simulink model "No_Guide_Experiments"  (R2020b)
settings: Solver=FixedStepAuto  StartTime=0.0  StopTime=1400  FixedStep=1  RelTol=1e-3  AbsTol=1e-6
model workspace (MATLAB code in the model file):
  | % load initial conditions and physical properties from file
  | 
  | data;
values from neighbouring files (symbols this model uses):
  c = 1005.4    [data.m]
  densAir = 1.2250    (= 1.225)    [data.m]
  M = (lenHouse*widHouse*htHouse+tan(pitRoof)*widHouse*lenHouse)*densAir    [data.m]
  Mdot = 60    [data.m]
  Req = RWall*RWindow/(RWall + RWindow)    [data.m]
libraries: dspnetwork x2
settings Model: ExtModeTrigMode=oneshot  ExtModeArmWhenConnect=off  ExtModeAutoUpdateStatusClock=off  OrderedModelArguments=off  Creator=The MathWorks, Inc.  LastModifiedBy=xinbo
settings SolverCC: AutoScaleAbsTol=off
settings DataIOCC: ExternalInput=[]  InitialState=[]  SaveFormat=Array  SaveOutput=off  SaveTime=off  SignalLoggingName=sldemo_househeat_output
settings OptimizationCC: BlockReduction=off  BooleanDataType=off  ExpressionDepthLimit=2147483647  InitFltsAndDblsToZero=on  LifeSpan=inf  BufferReusableBoundary=off
settings DebuggingCC: SaveWithParameterizedLinksMsg=none  UnderspecifiedInitializationDetection=Classic  MergeDetectMultiDrivingBlocksExec=none  SignalResolutionControl=TryResolveAllWithWarning  MultiTaskDSMMsg=warning  MultiTaskCondExecSysMsg=none  IntegerOverflowMsg=none  FcnCallInpInsideContextMsg=warning  BusObjectLabelMismatch=none  StateNameClashWarn=warning  SFUnexpectedBacktrackingDiag=warning  SFNoUnconditionalDefaultTransitionDiag=warning  SFExecutionAtInitializationDiag=none  IntegerSaturationMsg=none  ArithmeticOperatorsInVariantConditions=warning
settings HardwareCC: ProdBitPerPointer=32  ProdBitPerSizeT=32  ProdBitPerPtrDiffT=32  ProdLargestAtomicFloat=None  ProdIntDivRoundTo=Undefined  ProdEndianess=Unspecified  ProdWordSize=32  ProdHWDeviceType=32-bit Generic  TargetUnknown=on
settings ModelReferenceCC: PropagateSignalLabelsOutOfModel=off
settings SFSimCC: SimUseLocalCustomCode=off  CustomCodeUndefinedFunction=UseInterfaceOnly
settings RTWCC: RTWUseLocalCustomCode=off
settings CodeAppCC: StateflowObjectComments=on
settings GRTTargetCC: TargetFcnLib=ansi_tfl_tmw.mat  TargetLangStandard=C89/C90 (ANSI)  CombineOutputUpdateFcns=off  GRTInterface=on
settings ConfigComp: CovMetricSettings=dw  CovSaveCumulativeToWorkspaceVar=on  CovSaveSingleToWorkspaceVar=on  CovExternalEMLEnable=off

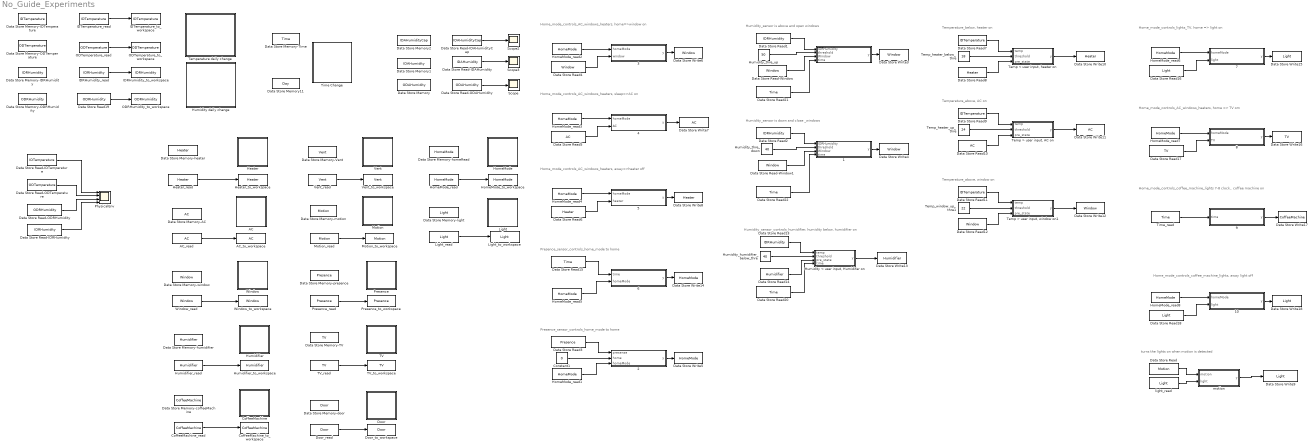
== system No_Guide_Experiments ==
  note: Home_mode_controls_coffee_machine_lights 7-8 clock,. coffee machine on
  note: Humidity_sensor is down and close _windows
  note: Home_mode_controls_AC_windows_heaters, home => TV om
  note: Temperature_below, heater on
  note: Home_mode_controls_lights_TV, home => light on
  note: Presence_sensor_controls_home_mode to home
  note: Presence_sensor_controls_home_mode to home
  note: Humidity_sensor_controls_humidifier, humidity below, humidifier on
  note: Temperature_above, window on
  note: Home_mode_controls_coffee_machine_lights, away light off
  note: Temperature_above, AC on
  note: Home_mode_controls_AC_windows_heaters, sleep=>AC on
  note: turns the lights on when motion is detected
  note: Home_mode_controls_AC_windows_heaters, away=>heater off
  note: Home_mode_controls_AC_windows_heaters, home=>window on
  note: Humidity_sensor is above and open windows
  " " : MATLAB Function  TreatAsAtomicUnit=on
  " 1" : MATLAB Function  TreatAsAtomicUnit=on
  " 10" : MATLAB Function  TreatAsAtomicUnit=on
  " 2" : MATLAB Function  TreatAsAtomicUnit=on
  " 3" : MATLAB Function  TreatAsAtomicUnit=on
  " 4" : MATLAB Function  TreatAsAtomicUnit=on
  " 5" : MATLAB Function  TreatAsAtomicUnit=on
  " 6" : MATLAB Function  TreatAsAtomicUnit=on
  " 7" : MATLAB Function  TreatAsAtomicUnit=on
  " 8" : MATLAB Function  TreatAsAtomicUnit=on
  " 9" : MATLAB Function  TreatAsAtomicUnit=on
  AC : Subsystem
      mask Display: image('$imagefile'); % Use "Edit Image" on toolstrip to change.
  AC_read : DataStoreRead  DataStoreName=AC
  AC_to_workspace : ToWorkspace  VariableName=AC  SampleTime=-1
      settings: Save2DSignal=2-D array (concatenate along first dimension)
  CoffeeMachine : Subsystem
      mask Display: image('$imagefile'); % Use "Edit Image" on toolstrip to change.
  CoffeeMachine_read : DataStoreRead  DataStoreName=CoffeeMachine
  CoffeeMachine_to_workspace : ToWorkspace  VariableName=CoffeeMachine  SampleTime=-1
      settings: Save2DSignal=2-D array (concatenate along first dimension)
  Constant1 : Constant  Value=0
  Data Store Memory11 : DataStoreMemory  DataStoreName=Day  ReadBeforeWriteMsg=warning  WriteAfterWriteMsg=warning  WriteAfterReadMsg=warning  ShowAdditionalParam=off  OutDataTypeStr=double
  Data Store Read : DataStoreRead  DataStoreName=Motion
  Data Store Read-IDAHumidity : DataStoreRead  DataStoreName=IDAHumidity
  Data Store Read-IDAHumidityCap : DataStoreRead  DataStoreName=IDAHumidityCap
  Data Store Read-IDRHumidity : DataStoreRead  DataStoreName=IDRHumidity
  Data Store Read-IDTemperature : DataStoreRead  DataStoreName=IDTemperature
  Data Store Read-ODAHumidity : DataStoreRead  DataStoreName=ODAHumidity
  Data Store Read-ODRHumidity : DataStoreRead  DataStoreName=ODRHumidity
  Data Store Read-ODTemperature : DataStoreRead  DataStoreName=ODTemperature
  Data Store Read1 : DataStoreRead  DataStoreName=IDRHumidity
  Data Store Read10 : DataStoreRead  DataStoreName=AC
  Data Store Read11 : DataStoreRead  DataStoreName=IDTemperature
  Data Store Read12 : DataStoreRead  DataStoreName=Window
  Data Store Read13 : DataStoreRead  DataStoreName=IDRHumidity
  Data Store Read14 : DataStoreRead  DataStoreName=Humidifier
  Data Store Read{15,20..22} (4 alike) : DataStoreRead  DataStoreName=Time
  Data Store Read16 : DataStoreRead  DataStoreName=Light
  Data Store Read17 : DataStoreRead  DataStoreName=TV
  Data Store Read18 : DataStoreRead  DataStoreName=Light
  Data Store Read19 : DataStoreRead  DataStoreName=ODRHumidity
  Data Store Read2 : DataStoreRead  DataStoreName=IDRHumidity
  Data Store Read3 : DataStoreRead  DataStoreName=Presence
  Data Store Read4 : DataStoreRead  DataStoreName=Window
  Data Store Read5 : DataStoreRead  DataStoreName=AC
  Data Store Read6 : DataStoreRead  DataStoreName=Heater
  Data Store Read7 : DataStoreRead  DataStoreName=IDTemperature
  Data Store Read8 : DataStoreRead  DataStoreName=Heater
  Data Store Read9 : DataStoreRead  DataStoreName=IDTemperature
  Data Store Write10 : DataStoreWrite  DataStoreName=Heater
  Data Store Write11 : DataStoreWrite  DataStoreName=AC
  Data Store Write{3..4,6,12} (4 alike) : DataStoreWrite  DataStoreName=Window
  Data Store Write13 : DataStoreWrite  DataStoreName=Humidifier
  Data Store Write14 : DataStoreWrite  DataStoreName=HomeMode
  Data Store Write15 : DataStoreWrite  DataStoreName=Light
  Data Store Write16 : DataStoreWrite  DataStoreName=TV
  Data Store Write17 : DataStoreWrite  DataStoreName=CoffeeMachine
  Data Store Write18 : DataStoreWrite  DataStoreName=Light
  Data Store Write5 : DataStoreWrite  DataStoreName=HomeMode
  Data Store Write7 : DataStoreWrite  DataStoreName=AC
  Data Store Write8 : DataStoreWrite  DataStoreName=Heater
  Data Store Write9 : DataStoreWrite  DataStoreName=Light
  Data Store Memory : DataStoreMemory  DataStoreName=ODAHumidity  ReadBeforeWriteMsg=warning  WriteAfterWriteMsg=warning  WriteAfterReadMsg=warning  ShowAdditionalParam=off
  Data Store Memory-AC : DataStoreMemory  DataStoreName=AC  ReadBeforeWriteMsg=warning  WriteAfterWriteMsg=warning  WriteAfterReadMsg=warning  ShowAdditionalParam=off  OutDataTypeStr=double
  Data Store Memory-IDRHumidity : DataStoreMemory  DataStoreName=IDRHumidity  ReadBeforeWriteMsg=warning  WriteAfterWriteMsg=warning  WriteAfterReadMsg=warning  InitialValue=80  ShowAdditionalParam=off  OutDataTypeStr=double
  Data Store Memory-IDTemperature : DataStoreMemory  DataStoreName=IDTemperature  ReadBeforeWriteMsg=warning  WriteAfterWriteMsg=warning  WriteAfterReadMsg=warning  InitialValue=25  ShowAdditionalParam=off  OutDataTypeStr=double
  Data Store Memory-ODRHumidity : DataStoreMemory  DataStoreName=ODRHumidity  ReadBeforeWriteMsg=warning  WriteAfterWriteMsg=warning  WriteAfterReadMsg=warning  InitialValue=45  ShowAdditionalParam=off  OutDataTypeStr=double
  Data Store Memory-ODTemperature : DataStoreMemory  DataStoreName=ODTemperature  ReadBeforeWriteMsg=warning  WriteAfterWriteMsg=warning  WriteAfterReadMsg=warning  ShowAdditionalParam=off  OutDataTypeStr=double
  Data Store Memory-TV : DataStoreMemory  DataStoreName=TV  ReadBeforeWriteMsg=warning  WriteAfterWriteMsg=warning  WriteAfterReadMsg=warning  ShowAdditionalParam=off  OutDataTypeStr=double
  Data Store Memory-Time : DataStoreMemory  DataStoreName=Time  ReadBeforeWriteMsg=warning  WriteAfterWriteMsg=warning  WriteAfterReadMsg=warning  ShowAdditionalParam=off  OutDataTypeStr=double
  Data Store Memory-Vent : DataStoreMemory  DataStoreName=Vent  ReadBeforeWriteMsg=warning  WriteAfterWriteMsg=warning  WriteAfterReadMsg=warning  ShowAdditionalParam=off
  Data Store Memory-coffeeMachine : DataStoreMemory  DataStoreName=CoffeeMachine  ReadBeforeWriteMsg=warning  WriteAfterWriteMsg=warning  WriteAfterReadMsg=warning  ShowAdditionalParam=off
  Data Store Memory-door : DataStoreMemory  DataStoreName=Door  ReadBeforeWriteMsg=warning  WriteAfterWriteMsg=warning  WriteAfterReadMsg=warning  ShowAdditionalParam=off  OutDataTypeStr=int8
  Data Store Memory-heater : DataStoreMemory  DataStoreName=Heater  ReadBeforeWriteMsg=warning  WriteAfterWriteMsg=warning  WriteAfterReadMsg=warning  ShowAdditionalParam=off
  Data Store Memory-homeRead : DataStoreMemory  DataStoreName=HomeMode  ReadBeforeWriteMsg=warning  WriteAfterWriteMsg=warning  WriteAfterReadMsg=warning  InitialValue=2  ShowAdditionalParam=off  OutDataTypeStr=double
  Data Store Memory-humidifier : DataStoreMemory  DataStoreName=Humidifier  ReadBeforeWriteMsg=warning  WriteAfterWriteMsg=warning  WriteAfterReadMsg=warning  ShowAdditionalParam=off
  Data Store Memory-light : DataStoreMemory  DataStoreName=Light  ReadBeforeWriteMsg=warning  WriteAfterWriteMsg=warning  WriteAfterReadMsg=warning  ShowAdditionalParam=off  OutDataTypeStr=double
  Data Store Memory-motion : DataStoreMemory  DataStoreName=Motion  ReadBeforeWriteMsg=warning  WriteAfterWriteMsg=warning  WriteAfterReadMsg=warning  ShowAdditionalParam=off
  Data Store Memory-presence : DataStoreMemory  DataStoreName=Presence  ReadBeforeWriteMsg=warning  WriteAfterWriteMsg=warning  WriteAfterReadMsg=warning  ShowAdditionalParam=off
  Data Store Memory-window : DataStoreMemory  DataStoreName=Window  ReadBeforeWriteMsg=warning  WriteAfterWriteMsg=warning  WriteAfterReadMsg=warning  ShowAdditionalParam=off
  Data Store Memory1 : DataStoreMemory  DataStoreName=IDAHumidity  ReadBeforeWriteMsg=warning  WriteAfterWriteMsg=warning  WriteAfterReadMsg=warning  ShowAdditionalParam=off
  Data Store Memory2 : DataStoreMemory  DataStoreName=IDAHumidityCap  ReadBeforeWriteMsg=warning  WriteAfterWriteMsg=warning  WriteAfterReadMsg=warning  ShowAdditionalParam=off
  Data Store Read-Window : DataStoreRead  DataStoreName=Window
  Data Store Read-Window1 : DataStoreRead  DataStoreName=Window
  Door : Subsystem
      mask Display: image('$imagefile'); % Use "Edit Image" on toolstrip to change.
  Door_read : DataStoreRead  DataStoreName=Door
  Door_to_workspace : ToWorkspace  VariableName=Door  SampleTime=-1
      settings: Save2DSignal=2-D array (concatenate along first dimension)
  Heater : Subsystem
      mask Display: image('$imagefile'); % Use "Edit Image" on toolstrip to change.
  Heater_read : DataStoreRead  DataStoreName=Heater
  Heater_to_workspace : ToWorkspace  VariableName=Heater  SampleTime=-1
      settings: Save2DSignal=2-D array (concatenate along first dimension)
  HomeMode : Subsystem
      mask Display: image('$imagefile'); % Use "Edit Image" on toolstrip to change.
  HomeMode_read{,1..8} (9 alike) : DataStoreRead  DataStoreName=HomeMode
  HomeMode_to_workspace : ToWorkspace  VariableName=HomeMode  SampleTime=-1
      settings: Save2DSignal=2-D array (concatenate along first dimension)
  Humidifier : Subsystem
      mask Display: image('$imagefile'); % Use "Edit Image" on toolstrip to change.
  Humidifier_read : DataStoreRead  DataStoreName=Humidifier
  Humidifier_to_workspace : ToWorkspace  VariableName=Humidifier  SampleTime=-1
      settings: Save2DSignal=2-D array (concatenate along first dimension)
  "Humidity < user input, Humidifer on" : MATLAB Function  TreatAsAtomicUnit=on
  Humidity daily change : Subsystem
      mask Display: image('$imagefile'); % Use "Edit Image" on toolstrip to change.
  Humidity_humidifier_below_thre : Constant  Value=40
  Humidity_thre_down : Constant  Value=40
  Humidity_thre_up : Constant  Value=50
  IDRHumidity_read : DataStoreRead  DataStoreName=IDRHumidity
  IDRHumidity_to_workspace : ToWorkspace  VariableName=IDRHumidity  SampleTime=-1
      settings: Save2DSignal=2-D array (concatenate along first dimension)
  IDTemperature_read : DataStoreRead  DataStoreName=IDTemperature
  IDTemperature_to_workspace : ToWorkspace  VariableName=IDTemperature  SampleTime=-1
      settings: Save2DSignal=2-D array (concatenate along first dimension)
  Light : Subsystem
      mask Display: image('$imagefile'); % Use "Edit Image" on toolstrip to change.
  Light_read : DataStoreRead  DataStoreName=Light
  Light_to_workspace : ToWorkspace  VariableName=Light  SampleTime=-1
      settings: Save2DSignal=2-D array (concatenate along first dimension)
  Motion : Subsystem
      mask Display: image('$imagefile'); % Use "Edit Image" on toolstrip to change.
  Motion_read : DataStoreRead  DataStoreName=Motion
  Motion_to_workspace : ToWorkspace  VariableName=Motion  SampleTime=-1
      settings: Save2DSignal=2-D array (concatenate along first dimension)
  ODRHumidity_to_workspace : ToWorkspace  VariableName=ODRHumidity  SampleTime=-1
      settings: Save2DSignal=2-D array (concatenate along first dimension)
  ODTemperature_read : DataStoreRead  DataStoreName=ODTemperature
  ODTemperature_to_workspace : ToWorkspace  VariableName=ODTemperature  SampleTime=-1
      settings: Save2DSignal=2-D array (concatenate along first dimension)
  PhysicalEnv : Scope  NumInputPorts=4
  Presence : Subsystem
      mask Display: image('$imagefile'); % Use "Edit Image" on toolstrip to change.
  Presence_read : DataStoreRead  DataStoreName=Presence
  Presence_to_workspace : ToWorkspace  VariableName=Presence  SampleTime=-1
      settings: Save2DSignal=2-D array (concatenate along first dimension)
  Scope : Scope
  Scope2 : Scope
  Scope3 : Scope
  TV : Subsystem
      mask Display: image('$imagefile'); % Use "Edit Image" on toolstrip to change.
  TV_read : DataStoreRead  DataStoreName=TV
  TV_to_workspace : ToWorkspace  VariableName=TV  SampleTime=-1
      settings: Save2DSignal=2-D array (concatenate along first dimension)
  "Temp < user input, heater on" : MATLAB Function  TreatAsAtomicUnit=on
  "Temp > user input, AC on" : MATLAB Function  TreatAsAtomicUnit=on
  "Temp > user input, window on1" : MATLAB Function  TreatAsAtomicUnit=on
  Temp_heater_below_thre : Constant  Value=18
  Temp_heater_up_thre : Constant  Value=24
  Temp_window_up_thre1 : Constant  Value=22
  Temperature daily change : Subsystem
      mask Display: image('$imagefile'); % Use "Edit Image" on toolstrip to change.
  Time Change : Subsystem
      mask Display: image('$imagefile'); % Use "Edit Image" on toolstrip to change.
  Time_read : DataStoreRead  DataStoreName=Time
  Vent : Subsystem
      mask Display: image('$imagefile'); % Use "Edit Image" on toolstrip to change.
  Vent_read : DataStoreRead  DataStoreName=Vent
  Vent_to_workspace : ToWorkspace  VariableName=Vent  SampleTime=-1
      settings: Save2DSignal=2-D array (concatenate along first dimension)
  Window : Subsystem
      mask Display: image('$imagefile'); % Use "Edit Image" on toolstrip to change.
  Window_read : DataStoreRead  DataStoreName=Window
  Window_to_workspace : ToWorkspace  VariableName=Window  SampleTime=-1
      settings: Save2DSignal=2-D array (concatenate along first dimension)
  light_read : DataStoreRead  DataStoreName=Light  SampleTime=1
  motion : MATLAB Function  TreatAsAtomicUnit=on
  wires:
  Temp_heater_up_thre/1 -> "Temp > user input, AC on"/2(threshold)
  Data Store Read21/1 -> " "/4(time)
  Data Store Read3/1 -> " 2"/1(presense)
  light_read/1 -> motion/2(light)
  " 10"/1(y) -> Data Store Write18/1
  motion/1(y) -> Data Store Write9/1
  " 4"/1(y) -> Data Store Write7/1
  Data Store Read-Window1/1 -> " 1"/3(Window)
  Humidity_thre_down/1 -> " 1"/2(threshold)
  HomeMode_read3/1 -> " 4"/1(homeMode)
  "Humidity < user input, Humidifer on"/1(y) -> Data Store Write13/1
  Data Store Read12/1 -> "Temp > user input, window on1"/3(pre_state)
  Data Store Read15/1 -> " 6"/1(time)
  " 2"/1(y) -> Data Store Write5/1
  HomeMode_read5/1 -> " 6"/2(homeMode)
  Data Store Read/1 -> motion/1(motion)
  Constant1/1 -> " 2"/2(home)
  Data Store Read6/1 -> " 5"/2(heater)
  Data Store Read11/1 -> "Temp > user input, window on1"/1(temp)
  " 5"/1(y) -> Data Store Write8/1
  Data Store Read16/1 -> " 7"/2(light)
  "Temp > user input, AC on"/1(y) -> Data Store Write11/1
  " "/1(y) -> Data Store Write3/1
  Data Store Read14/1 -> "Humidity < user input, Humidifer on"/3(pre_state)
  HomeMode_read4/1 -> " 5"/1(homeMode)
  HomeMode_read2/1 -> " 3"/1(homeMode)
  "Temp > user input, window on1"/1(y) -> Data Store Write12/1
  Data Store Read2/1 -> " 1"/1(IDRHumidity)
  HomeMode_read1/1 -> " 2"/3(homeMode)
  Data Store Read4/1 -> " 3"/2(window)
  Temp_heater_below_thre/1 -> "Temp < user input, heater on"/2(threshold)
  Data Store Read9/1 -> "Temp > user input, AC on"/1(temp)
  Temp_window_up_thre1/1 -> "Temp > user input, window on1"/2(threshold)
  " 3"/1(y) -> Data Store Write6/1
  Data Store Read1/1 -> " "/1(IDRHumidity)
  Data Store Read17/1 -> " 8"/2(TV)
  HomeMode_read6/1 -> " 7"/1(homeMode)
  Data Store Read7/1 -> "Temp < user input, heater on"/1(temp)
  Data Store Read10/1 -> "Temp > user input, AC on"/3(pre_state)
  HomeMode_read7/1 -> " 8"/1(homeMode)
  Time_read/1 -> " 9"/1(time)
  Data Store Read-Window/1 -> " "/3(Window)
  Data Store Read5/1 -> " 4"/2(AC)
  " 1"/1(y) -> Data Store Write4/1
  HomeMode_read8/1 -> " 10"/1(homeMode)
  Data Store Read8/1 -> "Temp < user input, heater on"/3(pre_state)
  "Temp < user input, heater on"/1(y) -> Data Store Write10/1
  Data Store Read13/1 -> "Humidity < user input, Humidifer on"/1(temp)
  Humidity_thre_up/1 -> " "/2(threshold)
  " 7"/1(y) -> Data Store Write15/1
  Data Store Read18/1 -> " 10"/2(light)
  " 9"/1(y) -> Data Store Write17/1
  " 8"/1(y) -> Data Store Write16/1
  Data Store Read20/1 -> "Humidity < user input, Humidifer on"/4(time)
  Humidity_humidifier_below_thre/1 -> "Humidity < user input, Humidifer on"/2(threshold)
  " 6"/1(y) -> Data Store Write14/1
  Data Store Read22/1 -> " 1"/4(time)
  Data Store Read-ODAHumidity/1 -> Scope/1
  Data Store Read-ODTemperature/1 -> PhysicalEnv/2
  Motion_read/1 -> Motion_to_workspace/1
  Data Store Read-IDRHumidity/1 -> PhysicalEnv/4
  Heater_read/1 -> Heater_to_workspace/1
  Vent_read/1 -> Vent_to_workspace/1
  Door_read/1 -> Door_to_workspace/1
  Data Store Read-IDTemperature/1 -> PhysicalEnv/1
  Window_read/1 -> Window_to_workspace/1
  Humidifier_read/1 -> Humidifier_to_workspace/1
  CoffeeMachine_read/1 -> CoffeeMachine_to_workspace/1
  IDRHumidity_read/1 -> IDRHumidity_to_workspace/1
  Data Store Read-IDAHumidityCap/1 -> Scope2/1
  Data Store Read-IDAHumidity/1 -> Scope3/1
  Data Store Read-ODRHumidity/1 -> PhysicalEnv/3
  Presence_read/1 -> Presence_to_workspace/1
  IDTemperature_read/1 -> IDTemperature_to_workspace/1
  TV_read/1 -> TV_to_workspace/1
  ODTemperature_read/1 -> ODTemperature_to_workspace/1
  Light_read/1 -> Light_to_workspace/1
  AC_read/1 -> AC_to_workspace/1
  Data Store Read19/1 -> ODRHumidity_to_workspace/1
  HomeMode_read/1 -> HomeMode_to_workspace/1

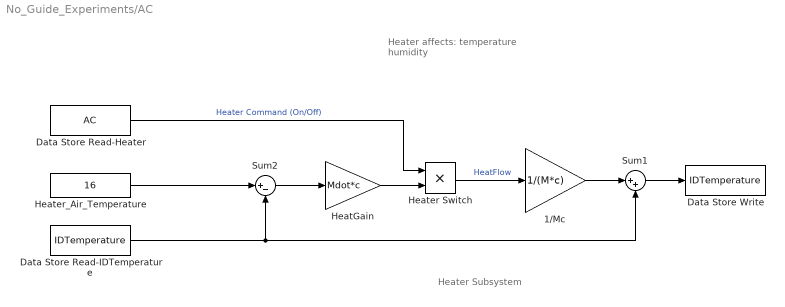
== system No_Guide_Experiments/AC ==
  note: Heater affects:
      | temperature
      | humidity
  note: Heater Subsystem
  1/Mc : Gain  Gain=1/(M*c)  SaturateOnIntegerOverflow=on  OutDataTypeStr=Inherit: Same as input  ParamDataTypeStr=Inherit: Same as input
  Data Store Read-Heater : DataStoreRead  DataStoreName=AC
  Data Store Read-IDTemperature : DataStoreRead  DataStoreName=IDTemperature
  Data Store Write : DataStoreWrite  DataStoreName=IDTemperature
  HeatGain : Gain  Gain=Mdot*c
  Heater Switch : Product  RndMeth=Zero
  Heater_Air_Temperature : Constant  Value=16
  Sum1 : Sum  Inputs=|++  InputSameDT=on  SaturateOnIntegerOverflow=on  OutDataTypeStr=Inherit: Same as first input
  Sum2 : Sum  Inputs=|+-
  wires:
  Data Store Read-Heater/1 -> Heater Switch/1  "Heater Command (On/Off)"
  Sum2/1 -> HeatGain/1
  Heater_Air_Temperature/1 -> Sum2/1
  HeatGain/1 -> Heater Switch/2
  Heater Switch/1 -> 1/Mc/1  "HeatFlow"
  1/Mc/1 -> Sum1/1
  Data Store Read-IDTemperature/1 -> Sum1/2, Sum2/2
  Sum1/1 -> Data Store Write/1

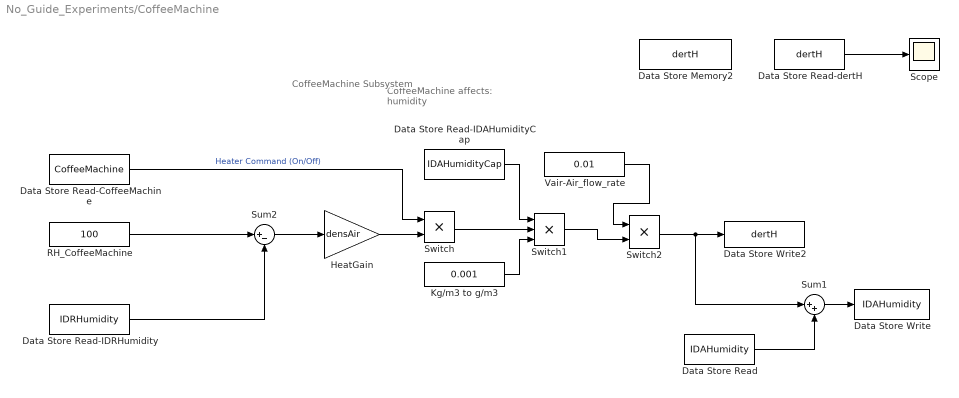
== system No_Guide_Experiments/CoffeeMachine ==
  note: CoffeeMachine affects:
      | humidity
  note: CoffeeMachine
      |  Subsystem
  " Switch" : Product  RndMeth=Zero
  " Switch1" : Product  Inputs=3  RndMeth=Zero
  " Switch2" : Product  RndMeth=Zero
  Data Store Read : DataStoreRead  DataStoreName=IDAHumidity
  Data Store Read-CoffeeMachine : DataStoreRead  DataStoreName=CoffeeMachine
  Data Store Read-IDAHumidityCap : DataStoreRead  DataStoreName=IDAHumidityCap
  Data Store Read-IDRHumidity : DataStoreRead  DataStoreName=IDRHumidity
  Data Store Read-dertH : DataStoreRead  DataStoreName=dertH
  Data Store Write : DataStoreWrite  DataStoreName=IDAHumidity
  Data Store Write2 : DataStoreWrite  DataStoreName=dertH
  Data Store Memory2 : DataStoreMemory  DataStoreName=dertH  ReadBeforeWriteMsg=warning  WriteAfterWriteMsg=warning  WriteAfterReadMsg=warning  ShowAdditionalParam=off
  HeatGain : Gain  Gain=densAir
  Kg/m3 to g/m3 : Constant  Value=0.001
  RH_CoffeeMachine : Constant  Value=100
  Scope : Scope
  Sum1 : Sum  Inputs=|++
  Sum2 : Sum  Inputs=|+-
  Vair-Air_flow_rate : Constant  Value=0.01
  wires:
  Data Store Read-CoffeeMachine/1 -> " Switch"/1  "Heater Command (On/Off)"
  Sum2/1 -> HeatGain/1
  RH_CoffeeMachine/1 -> Sum2/1
  HeatGain/1 -> " Switch"/2
  " Switch"/1 -> " Switch1"/2
  Data Store Read-IDRHumidity/1 -> Sum2/2
  Data Store Read-IDAHumidityCap/1 -> " Switch1"/1
  Kg/m3 to g/m3/1 -> " Switch1"/3
  " Switch1"/1 -> " Switch2"/2
  Vair-Air_flow_rate/1 -> " Switch2"/1
  " Switch2"/1 -> Sum1/1, Data Store Write2/1
  Sum1/1 -> Data Store Write/1
  Data Store Read-dertH/1 -> Scope/1
  Data Store Read/1 -> Sum1/2

== system No_Guide_Experiments/Door ==

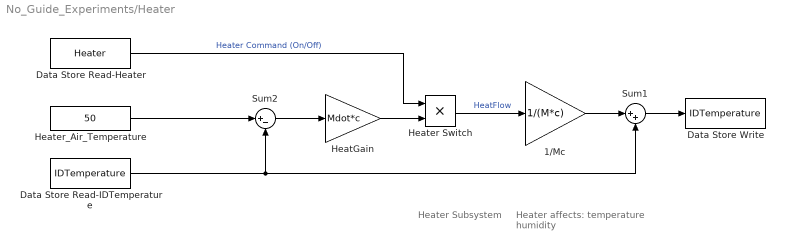
== system No_Guide_Experiments/Heater ==
  note: Heater affects:
      | temperature
      | humidity
  note: Heater Subsystem
  1/Mc : Gain  Gain=1/(M*c)  SaturateOnIntegerOverflow=on  OutDataTypeStr=Inherit: Same as input  ParamDataTypeStr=Inherit: Same as input
  Data Store Read-Heater : DataStoreRead  DataStoreName=Heater
  Data Store Read-IDTemperature : DataStoreRead  DataStoreName=IDTemperature
  Data Store Write : DataStoreWrite  DataStoreName=IDTemperature
  HeatGain : Gain  Gain=Mdot*c
  Heater Switch : Product  RndMeth=Zero
  Heater_Air_Temperature : Constant  Value=50
  Sum1 : Sum  Inputs=|++  InputSameDT=on  SaturateOnIntegerOverflow=on  OutDataTypeStr=Inherit: Same as first input
  Sum2 : Sum  Inputs=|+-
  wires:
  Data Store Read-Heater/1 -> Heater Switch/1  "Heater Command (On/Off)"
  Sum2/1 -> HeatGain/1
  Heater_Air_Temperature/1 -> Sum2/1
  HeatGain/1 -> Heater Switch/2
  Heater Switch/1 -> 1/Mc/1  "HeatFlow"
  1/Mc/1 -> Sum1/1
  Data Store Read-IDTemperature/1 -> Sum1/2, Sum2/2
  Sum1/1 -> Data Store Write/1

== system No_Guide_Experiments/HomeMode ==

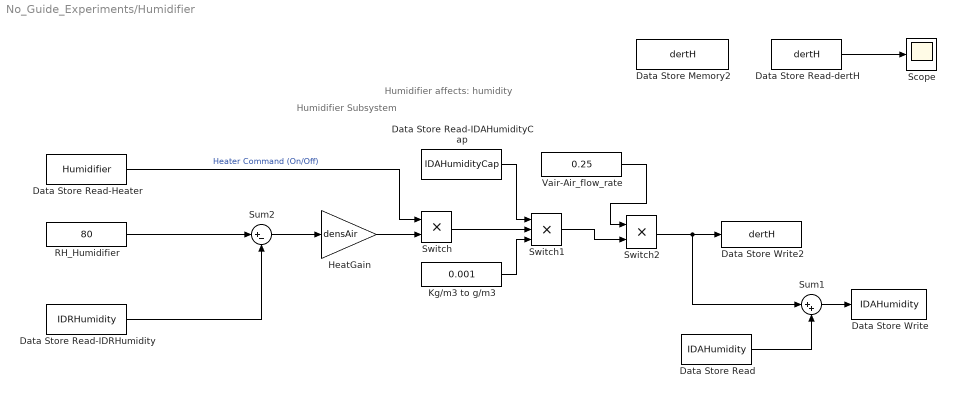
== system No_Guide_Experiments/Humidifier ==
  note: Humidifier affects:
      | humidity
  note: Humidifier
      |  Subsystem
  " Switch" : Product  RndMeth=Zero
  " Switch1" : Product  Inputs=3  RndMeth=Zero
  " Switch2" : Product  RndMeth=Zero
  Data Store Read : DataStoreRead  DataStoreName=IDAHumidity
  Data Store Read-Heater : DataStoreRead  DataStoreName=Humidifier
  Data Store Read-IDAHumidityCap : DataStoreRead  DataStoreName=IDAHumidityCap
  Data Store Read-IDRHumidity : DataStoreRead  DataStoreName=IDRHumidity
  Data Store Read-dertH : DataStoreRead  DataStoreName=dertH
  Data Store Write : DataStoreWrite  DataStoreName=IDAHumidity
  Data Store Write2 : DataStoreWrite  DataStoreName=dertH
  Data Store Memory2 : DataStoreMemory  DataStoreName=dertH  ReadBeforeWriteMsg=warning  WriteAfterWriteMsg=warning  WriteAfterReadMsg=warning  ShowAdditionalParam=off
  HeatGain : Gain  Gain=densAir
  Kg/m3 to g/m3 : Constant  Value=0.001
  RH_Humidifier : Constant  Value=80
  Scope : Scope
  Sum1 : Sum  Inputs=|++
  Sum2 : Sum  Inputs=|+-
  Vair-Air_flow_rate : Constant  Value=0.25
  wires:
  Data Store Read-Heater/1 -> " Switch"/1  "Heater Command (On/Off)"
  Sum2/1 -> HeatGain/1
  RH_Humidifier/1 -> Sum2/1
  HeatGain/1 -> " Switch"/2
  " Switch"/1 -> " Switch1"/2
  Data Store Read-IDRHumidity/1 -> Sum2/2
  Data Store Read-IDAHumidityCap/1 -> " Switch1"/1
  Kg/m3 to g/m3/1 -> " Switch1"/3
  " Switch1"/1 -> " Switch2"/2
  Vair-Air_flow_rate/1 -> " Switch2"/1
  " Switch2"/1 -> Sum1/1, Data Store Write2/1
  Sum1/1 -> Data Store Write/1
  Data Store Read-dertH/1 -> Scope/1
  Data Store Read/1 -> Sum1/2

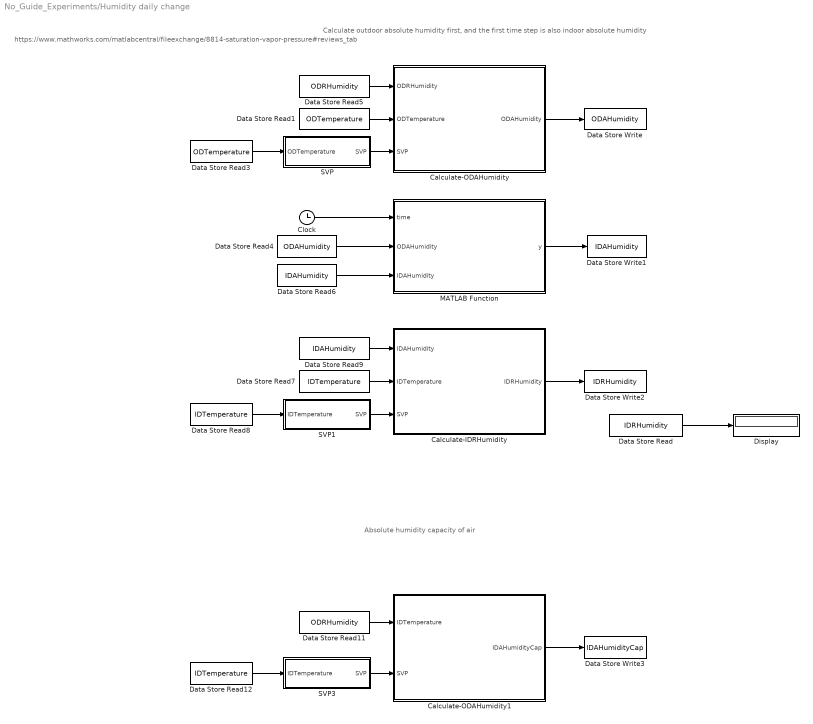
== system No_Guide_Experiments/Humidity daily change ==
  note: Absolute humidity capacity of air
  note: https://www.mathworks.com/matlabcentral/fileexchange/8814-saturation-vapor-pressure#reviews_tab
  note: Calculate outdoor absolute humidity first, and the first time step is also indoor absolute humidity
  Calculate-IDRHumidity : MATLAB Function  TreatAsAtomicUnit=on
  Calculate-ODAHumidity : MATLAB Function  TreatAsAtomicUnit=on
  Calculate-ODAHumidity1 : MATLAB Function  TreatAsAtomicUnit=on
  Clock : Clock
  Data Store Read : DataStoreRead  DataStoreName=IDRHumidity
  Data Store Read1 : DataStoreRead  DataStoreName=ODTemperature
  Data Store Read11 : DataStoreRead  DataStoreName=ODRHumidity
  Data Store Read12 : DataStoreRead  DataStoreName=IDTemperature
  Data Store Read3 : DataStoreRead  DataStoreName=ODTemperature
  Data Store Read4 : DataStoreRead  DataStoreName=ODAHumidity
  Data Store Read5 : DataStoreRead  DataStoreName=ODRHumidity
  Data Store Read6 : DataStoreRead  DataStoreName=IDAHumidity
  Data Store Read7 : DataStoreRead  DataStoreName=IDTemperature
  Data Store Read8 : DataStoreRead  DataStoreName=IDTemperature
  Data Store Read9 : DataStoreRead  DataStoreName=IDAHumidity
  Data Store Write : DataStoreWrite  DataStoreName=ODAHumidity
  Data Store Write1 : DataStoreWrite  DataStoreName=IDAHumidity
  Data Store Write2 : DataStoreWrite  DataStoreName=IDRHumidity
  Data Store Write3 : DataStoreWrite  DataStoreName=IDAHumidityCap
  Display : Display
  MATLAB Function : MATLAB Function  TreatAsAtomicUnit=on
  SVP : MATLAB Function  TreatAsAtomicUnit=on
  SVP1 : MATLAB Function  TreatAsAtomicUnit=on
  SVP3 : MATLAB Function  TreatAsAtomicUnit=on
  wires:
  Data Store Read3/1 -> SVP/1(ODTemperature)
  Data Store Read5/1 -> Calculate-ODAHumidity/1(ODRHumidity)
  SVP/1(SVP) -> Calculate-ODAHumidity/3(SVP)
  Data Store Read1/1 -> Calculate-ODAHumidity/2(ODTemperature)
  Calculate-ODAHumidity/1(ODAHumidity) -> Data Store Write/1
  Clock/1 -> MATLAB Function/1(time)
  Data Store Read4/1 -> MATLAB Function/2(ODAHumidity)
  MATLAB Function/1(y) -> Data Store Write1/1
  Data Store Read6/1 -> MATLAB Function/3(IDAHumidity)
  Calculate-IDRHumidity/1(IDRHumidity) -> Data Store Write2/1
  SVP1/1(SVP) -> Calculate-IDRHumidity/3(SVP)
  Data Store Read9/1 -> Calculate-IDRHumidity/1(IDAHumidity)
  Data Store Read8/1 -> SVP1/1(IDTemperature)
  Data Store Read7/1 -> Calculate-IDRHumidity/2(IDTemperature)
  Data Store Read11/1 -> Calculate-ODAHumidity1/1(IDTemperature)
  Calculate-ODAHumidity1/1(IDAHumidityCap) -> Data Store Write3/1
  SVP3/1(SVP) -> Calculate-ODAHumidity1/2(SVP)
  Data Store Read12/1 -> SVP3/1(IDTemperature)
  Data Store Read/1 -> Display/1

== system No_Guide_Experiments/Light ==

== system No_Guide_Experiments/Motion ==

== system No_Guide_Experiments/Presence ==

== system No_Guide_Experiments/TV ==

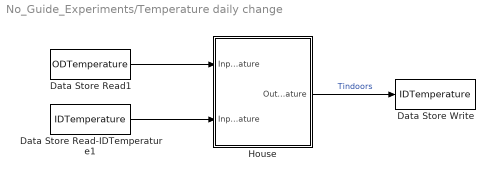
== system No_Guide_Experiments/Temperature daily change ==
  Data Store Read-IDTemperature1 : DataStoreRead  DataStoreName=IDTemperature
  Data Store Read1 : DataStoreRead  DataStoreName=ODTemperature
  Data Store Write : DataStoreWrite  DataStoreName=IDTemperature
  House : Subsystem
      mask Display: image('/Users/xinbo/E/paper3/program_clean/digital_twin/images/home.png'); % Use "Edit Image" on toolstrip to change.
  wires:
  Data Store Read-IDTemperature1/1 -> House/2(Input-IDTemperature)
  Data Store Read1/1 -> House/1(Input-ODTemperature)
  House/1(Output-IDTemperature) -> Data Store Write/1  "Tindoors"

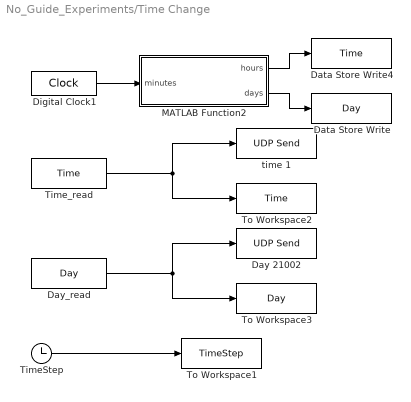
== system No_Guide_Experiments/Time Change ==
  Data Store Write : DataStoreWrite  DataStoreName=Day
  Data Store Write4 : DataStoreWrite  DataStoreName=Time  SampleTime=1
  Day 21002 : dspnetwork/UDP Send  remoteURL='127.0.0.1'  remotePort=21002  localURL='0.0.0.0'  localPortSource=Automatically determine  localPort=-1  sendBufferSize=8192  sampletime=-1  blockPlatform=[]  separateLengthPort=0
  Day_read : DataStoreRead  DataStoreName=Day
  Digital Clock1 : DigitalClock
  MATLAB Function2 : MATLAB Function  TreatAsAtomicUnit=on
  TimeStep : Clock
  Time_read : DataStoreRead  DataStoreName=Time  SampleTime=1
  To Workspace1 : ToWorkspace  VariableName=TimeStep  SampleTime=-1
      settings: Save2DSignal=2-D array (concatenate along first dimension)
  To Workspace2 : ToWorkspace  VariableName=Time  SampleTime=-1
  To Workspace3 : ToWorkspace  VariableName=Day  SampleTime=-1
  time 1 : dspnetwork/UDP Send  remoteURL='127.0.0.1'  remotePort=21001  localURL='0.0.0.0'  localPortSource=Automatically determine  localPort=-1  sendBufferSize=8192  sampletime=-1  blockPlatform=[]  separateLengthPort=0
  wires:
  MATLAB Function2/2(days) -> Data Store Write/1
  MATLAB Function2/1(hours) -> Data Store Write4/1
  Time_read/1 -> time 1/1, To Workspace2/1
  Day_read/1 -> Day 21002/1, To Workspace3/1
  Digital Clock1/1 -> MATLAB Function2/1(minutes)
  TimeStep/1 -> To Workspace1/1

== system No_Guide_Experiments/Vent ==

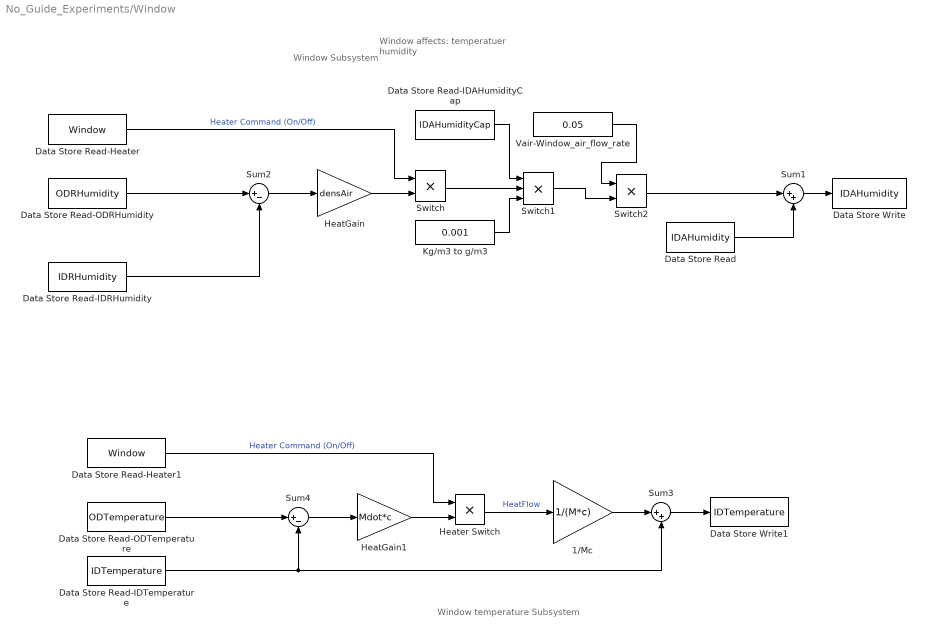
== system No_Guide_Experiments/Window ==
  note: Window
      |  Subsystem
  note: Window affects:
      | temperatuer
      | humidity
  note: Window temperature Subsystem
  " Switch" : Product  RndMeth=Zero
  " Switch1" : Product  Inputs=3  RndMeth=Zero
  " Switch2" : Product  RndMeth=Zero
  1/Mc : Gain  Gain=1/(M*c)  SaturateOnIntegerOverflow=on  OutDataTypeStr=Inherit: Same as input  ParamDataTypeStr=Inherit: Same as input
  Data Store Read : DataStoreRead  DataStoreName=IDAHumidity
  Data Store Read-Heater : DataStoreRead  DataStoreName=Window
  Data Store Read-Heater1 : DataStoreRead  DataStoreName=Window
  Data Store Read-IDAHumidityCap : DataStoreRead  DataStoreName=IDAHumidityCap
  Data Store Read-IDRHumidity : DataStoreRead  DataStoreName=IDRHumidity
  Data Store Read-IDTemperature : DataStoreRead  DataStoreName=IDTemperature
  Data Store Read-ODRHumidity : DataStoreRead  DataStoreName=ODRHumidity
  Data Store Read-ODTemperature : DataStoreRead  DataStoreName=ODTemperature
  Data Store Write : DataStoreWrite  DataStoreName=IDAHumidity
  Data Store Write1 : DataStoreWrite  DataStoreName=IDTemperature
  HeatGain : Gain  Gain=densAir
  HeatGain1 : Gain  Gain=Mdot*c
  Heater Switch : Product  RndMeth=Zero
  Kg/m3 to g/m3 : Constant  Value=0.001
  Sum1 : Sum  Inputs=|++
  Sum2 : Sum  Inputs=|+-
  Sum3 : Sum  Inputs=|++  InputSameDT=on  SaturateOnIntegerOverflow=on  OutDataTypeStr=Inherit: Same as first input
  Sum4 : Sum  Inputs=|+-
  Vair-Window_air_flow_rate : Constant  Value=0.05
  wires:
  Vair-Window_air_flow_rate/1 -> " Switch2"/1
  Kg/m3 to g/m3/1 -> " Switch1"/3
  HeatGain/1 -> " Switch"/2
  Sum1/1 -> Data Store Write/1
  " Switch"/1 -> " Switch1"/2
  Data Store Read-ODRHumidity/1 -> Sum2/1
  Data Store Read-IDAHumidityCap/1 -> " Switch1"/1
  " Switch1"/1 -> " Switch2"/2
  Data Store Read-IDRHumidity/1 -> Sum2/2
  " Switch2"/1 -> Sum1/1
  Data Store Read-Heater/1 -> " Switch"/1  "Heater Command (On/Off)"
  Data Store Read/1 -> Sum1/2
  Sum2/1 -> HeatGain/1
  Data Store Read-ODTemperature/1 -> Sum4/1
  Sum4/1 -> HeatGain1/1
  HeatGain1/1 -> Heater Switch/2
  Data Store Read-Heater1/1 -> Heater Switch/1  "Heater Command (On/Off)"
  1/Mc/1 -> Sum3/1
  Sum3/1 -> Data Store Write1/1
  Data Store Read-IDTemperature/1 -> Sum3/2, Sum4/2
  Heater Switch/1 -> 1/Mc/1  "HeatFlow"

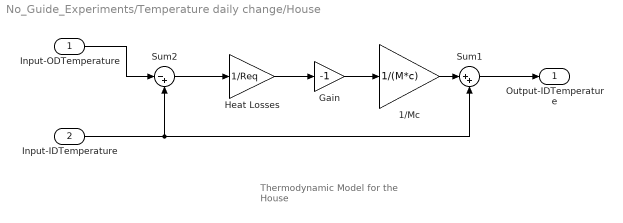
== system No_Guide_Experiments/Temperature daily change/House ==
  note: Thermodynamic Model
      | for the House
  Input-ODTemperature : Inport
  Input-IDTemperature : Inport  Port=2
  1/Mc : Gain  Gain=1/(M*c)  SaturateOnIntegerOverflow=on  OutDataTypeStr=Inherit: Same as input  ParamDataTypeStr=Inherit: Same as input
  Gain : Gain  Gain=-1
  Heat Losses : Gain  Gain=1/Req  SaturateOnIntegerOverflow=on  OutDataTypeStr=Inherit: Same as input  ParamDataTypeStr=Inherit: Same as input
  Sum1 : Sum  Inputs=|++  InputSameDT=on  SaturateOnIntegerOverflow=on  OutDataTypeStr=Inherit: Same as first input
  Sum2 : Sum  Inputs=|-+  InputSameDT=on  SaturateOnIntegerOverflow=on  OutDataTypeStr=Inherit: Same as first input
  Output-IDTemperature : Outport  InitialOutput=0  VectorParamsAs1DForOutWhenUnconnected=off
  wires:
  Input-ODTemperature/1 -> Sum2/1
  Gain/1 -> 1/Mc/1
  Sum2/1 -> Heat Losses/1
  Heat Losses/1 -> Gain/1
  1/Mc/1 -> Sum1/1
  Sum1/1 -> Output-IDTemperature/1
  Input-IDTemperature/1 -> Sum1/2, Sum2/2

== matlab function No_Guide_Experiments/ 4 ==
  data: homeMode input; AC input; y output
function y = ST11(homeMode, AC)

if(homeMode == 1)
    y = 1;
else
    y = AC;
end

== matlab function No_Guide_Experiments/ 5 ==
  data: homeMode input; heater input; y output
function y = ST11(homeMode, heater)

if(homeMode == 2)
    y = 0;
else
    y = heater;
end

== matlab function No_Guide_Experiments/motion ==
  data: motion input; y output; light input
function y= motionMode(motion,light)

if(motion == 1)
    y = 1;
else
    y = light;
end

== matlab function No_Guide_Experiments/Humidity daily change/MATLAB Function ==
  data: time input; y output; ODAHumidity input; IDAHumidity input
function y = CalIDAHumidity(time, ODAHumidity, IDAHumidity)

if(time == 0)
    y = ODAHumidity;
else
    y = IDAHumidity;
end

== matlab function No_Guide_Experiments/Temp > user input, AC on ==
  data: temp input; y output; threshold input; pre_state input
function y = ST11(temp, threshold, pre_state)

if(temp > threshold)
    y = 1;
else
    y = pre_state;
end

== matlab function No_Guide_Experiments/Temp < user input, heater on ==
  data: temp input; y output; threshold input; pre_state input
function y = ST11(temp, threshold, pre_state)

if(temp < threshold)
    y = 1;
else
    y = pre_state;
end

== matlab function No_Guide_Experiments/Temp > user input, window on1 ==
  data: temp input; y output; threshold input; pre_state input
function y = ST11(temp, threshold, pre_state)

if(temp > threshold)
    y = 1;
else
    y = pre_state;
end

== matlab function No_Guide_Experiments/Humidity < user input, Humidifer on ==
  data: temp input; y output; threshold input; pre_state input; time input
function y = ST11(temp, threshold, pre_state, time)

if(temp < threshold && time > 0)
    y = 1;
else
    y = pre_state;
end

== matlab function No_Guide_Experiments/Time Change/MATLAB Function2 ==
  data: minutes input; hours output; days output
function [hours, days]= calTime(minutes)

hours = minutes/60;
days = 0;

while(hours > 24)
    hours = hours - 24;
    days = days + 1;
end

== matlab function No_Guide_Experiments/ 6 ==
  data: time input; y output; homeMode input
function y = ST11(time, homeMode)

if(time > 18 && time <23)
    y = 0;
elseif (time >23 || time < 6)
    y = 1;
elseif (time > 8 && time < 18)
    y = 2;
else
    y = homeMode;
end

== matlab function No_Guide_Experiments/ 7 ==
  data: homeMode input; light input; y output
function y = ST11(homeMode, light)

if(homeMode == 0)
    y = 1;
else
    y = light;
end

== matlab function No_Guide_Experiments/ 8 ==
  data: homeMode input; TV input; y output
function y = ST11(homeMode, TV)

if(homeMode == 1)
    y = 1;
else
    y = TV;
end

== matlab function No_Guide_Experiments/ 10 ==
  data: homeMode input; light input; y output
function y = ST11(homeMode, light)

if(homeMode == 2)
    y = 0;
else
    y = light;
end

== matlab function No_Guide_Experiments/ 9 ==
  data: time input; y output
function y = ST11(time)

if(time > 7 && time < 8)
    y = 1;
else
    y = 0;
end

== matlab function No_Guide_Experiments/Humidity daily change/SVP ==
  data: SVP output; ODTemperature input
function SVP = svp(ODTemperature)

% [°C] = [K] - 273.15
% https://www.mathworks.com/matlabcentral/fileexchange/8814-saturation-vapor-pressure
% T = temperature on Kelvin scale
% SVP = saturation vapor pressure according to Goff & Gratch Equation (1946)
% SVP in Pascal

Ts = 373.15;    % standard temperature at steam point on Kelvin scale (Goff, 1965)
Ps = 101324.6;  % standard atmospheric pressure at steam point (Pascal)

T = ODTemperature + 273.15;
log10SVP = -7.90298*(Ts./T - 1) + 5.02808*log10(Ts./T) -1.3816e-7*(10.^(11.344*(1 - T./Ts)) - 1) + 8.1328e-3*(10.^(3.49149*(1 - Ts./T)) - 1) + log10(Ps);

SVP = 10.^(log10SVP);

== matlab function No_Guide_Experiments/Humidity daily change/Calculate-IDRHumidity ==
  data: IDRHumidity output; IDAHumidity input; IDTemperature input; SVP input
function IDRHumidity = CalIDRHumidity(IDAHumidity, IDTemperature, SVP)

% https://www.mathworks.com/matlabcentral/fileexchange/8814-saturation-vapor-pressure

% ODTemperature in Celius
% [°C] = [K] - 273.15
% SVP = saturation vapor pressure according to Goff & Gratch Equation (1946)
% SVP in Pascal
% IDAHumidity is in kg/m3, absolute humidity


Rw = 461.5;
% J/(kg*K) Rw is specific gas constant for water vapor 
IDTemperature = IDTemperature + 273.15;

IDRHumidity = IDAHumidity * Rw * IDTemperature * 100 / SVP;

if (IDRHumidity > 100)
    IDRHumidity = 100;
end

== matlab function No_Guide_Experiments/Humidity daily change/Calculate-ODAHumidity ==
  data: ODAHumidity output; ODRHumidity input; ODTemperature input; SVP input
function ODAHumidity = CalODAHumidity(ODRHumidity, ODTemperature, SVP)

% https://www.mathworks.com/matlabcentral/fileexchange/8814-saturation-vapor-pressure

% ODTemperature in Celius
% [°C] = [K] - 273.15
% SVP = saturation vapor pressure according to Goff & Gratch Equation (1946)
% SVP in Pascal
% ODAHumidity is in kg/m3

Rw = 461.5;
% J/(kg*K) Rw is specific gas constant for water vapor 
T = ODTemperature + 273.15;
ODAHumidity = ODRHumidity * SVP / (Rw * T * 100);

== matlab function No_Guide_Experiments/Humidity daily change/SVP1 ==
  data: SVP output; IDTemperature input
function SVP = svp(IDTemperature)

% [°C] = [K] - 273.15
% https://www.mathworks.com/matlabcentral/fileexchange/8814-saturation-vapor-pressure
% T = temperature on Kelvin scale
% SVP = saturation vapor pressure according to Goff & Gratch Equation (1946)
% SVP in Pascal

Ts = 373.15;    % standard temperature at steam point on Kelvin scale (Goff, 1965)
Ps = 101324.6;  % standard atmospheric pressure at steam point (Pascal)

T = IDTemperature + 273.15;
log10SVP = -7.90298*(Ts./T - 1) + 5.02808*log10(Ts./T) -1.3816e-7*(10.^(11.344*(1 - T./Ts)) - 1) + 8.1328e-3*(10.^(3.49149*(1 - Ts./T)) - 1) + log10(Ps);

SVP = 10.^(log10SVP);

== matlab function No_Guide_Experiments/Humidity daily change/Calculate-ODAHumidity1 ==
  data: IDAHumidityCap output; IDTemperature input; SVP input
function IDAHumidityCap = CalIDAHumidityCap(IDTemperature, SVP)

% https://www.mathworks.com/matlabcentral/fileexchange/8814-saturation-vapor-pressure

% ODTemperature in Celius
% [°C] = [K] - 273.15
% SVP = saturation vapor pressure according to Goff & Gratch Equation (1946)
% SVP in Pascal
% AHumidity is in kg/m3

Rw = 461.5;
% J/(kg*K) Rw is specific gas constant for water vapor 
T = IDTemperature + 273.15;
IDRHumidityCap = 100;
IDAHumidityCap = IDRHumidityCap * SVP / (Rw * T * 100);

== matlab function No_Guide_Experiments/  ==
  data: IDRHumidity input; y output; threshold input; Window input; time input
function y = ST1(IDRHumidity, threshold, Window, time)

if(IDRHumidity > threshold && time > 0)
    y = 1;
else
    y = Window;
end

== matlab function No_Guide_Experiments/Humidity daily change/SVP3 ==
  data: SVP output; IDTemperature input
function SVP = svp(IDTemperature)

% [°C] = [K] - 273.15
% https://www.mathworks.com/matlabcentral/fileexchange/8814-saturation-vapor-pressure
% T = temperature on Kelvin scale
% SVP = saturation vapor pressure according to Goff & Gratch Equation (1946)
% SVP in Pascal

Ts = 373.15;    % standard temperature at steam point on Kelvin scale (Goff, 1965)
Ps = 101324.6;  % standard atmospheric pressure at steam point (Pascal)

T = IDTemperature + 273.15;
log10SVP = -7.90298*(Ts./T - 1) + 5.02808*log10(Ts./T) -1.3816e-7*(10.^(11.344*(1 - T./Ts)) - 1) + 8.1328e-3*(10.^(3.49149*(1 - Ts./T)) - 1) + log10(Ps);

SVP = 10.^(log10SVP);

== matlab function No_Guide_Experiments/ 1 ==
  data: IDRHumidity input; y output; threshold input; Window input; time input
function y = ST1(IDRHumidity, threshold, Window, time)

if(IDRHumidity < threshold && time > 0)
    y = 0;
else
    y = Window;
end

== matlab function No_Guide_Experiments/ 2 ==
  data: presense input; y output; home input; homeMode input
function y = ST11(presense, home, homeMode)

if(presense > 0)
    y = home;
else
    y = homeMode;
end

== matlab function No_Guide_Experiments/ 3 ==
  data: homeMode input; window input; y output
function y = ST11(homeMode, window)

if(homeMode == 0)
    y = 1;
else
    y = window;
end
